simulink model "simple_high_fidelity_tilting_quadrotor_test"  (R2022b)
settings: Solver=ode4  StartTime=0.0  StopTime=10.0  FixedStep=T_s  RelTol=1e-3
undefined symbols (not defined in the file): alpha_0, N, w_bar_0
libraries: slpidlib x2, uavutilslib x1
settings Model: PauseTimes=0.2  Creator=pozzan  LastModifiedBy=pozzan

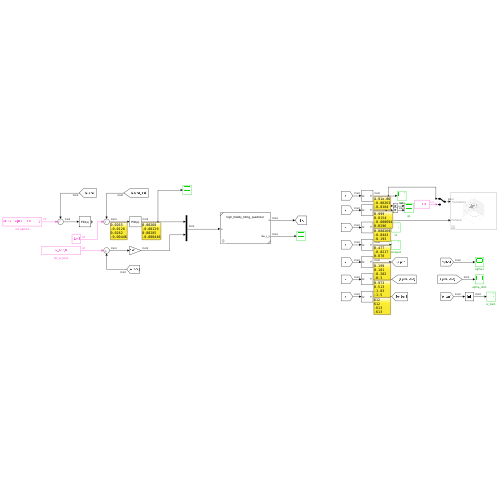
[thumbnail: Simulink's stored preview of the top-level diagram]
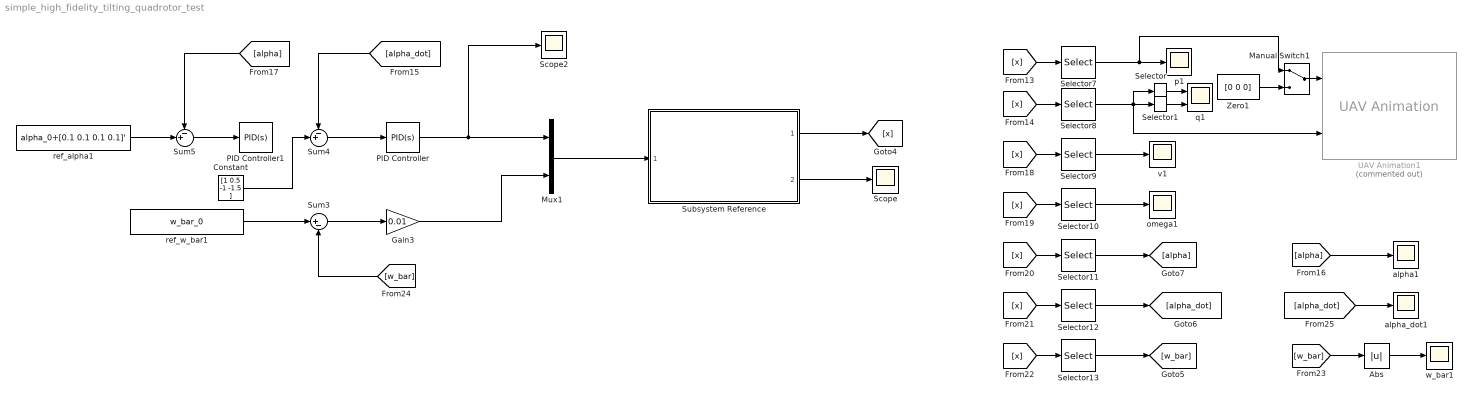
== system simple_high_fidelity_tilting_quadrotor_test ==
  Abs : Abs  SaturateOnIntegerOverflow=off
  Constant : Constant  Value=[1 0.5 -1 -1.5 ]
  Gain3 : Gain  Gain=0.01
  Manual Switch1 : ManualSwitch
  Mux1 : Mux  Inputs=2
  PID Controller : slpidlib/PID Controller  Controller=PID  Form=Parallel  TimeDomain=Continuous-time  UseExternalTs=off  SampleTime=-1  IntegratorMethod=Forward Euler  FilterMethod=Forward Euler  ControllerParametersSource=internal  P=0.1  I=0  UseKiTs=off  D=0.0001  N=100  UseFilter=on  TunerSelectOption=Transfer Function Based (PID Tuner App)  InitialConditionSource=internal  InitialConditionForIntegrator=0  InitialConditionForFilter=0  DifferentiatorICPrevScaledInput=0  ExternalReset=none  TrackingMode=off  Kt=1  LimitOutput=off  SatLimitsSource=internal  UpperSaturationLimit=inf  LowerSaturationLimit=-inf  LinearizeAsGain=on  AntiWindupMode=none  Kb=1  LimitIntegrator=off  UpperIntegratorSaturationLimit=inf  LowerIntegratorSaturationLimit=-inf  POutMin=[]  POutMax=[]  IOutMin=[]  IOutMax=[]  DOutMin=[]  DOutMax=[]  NOutMin=[]  NOutMax=[]  SumOutMin=[]  SumOutMax=[]  SaturationOutMin=[]  SaturationOutMax=[]  PParamMin=[]  PParamMax=[]  IParamMin=[]  IParamMax=[]  DParamMin=[]  DParamMax=[]  NParamMin=[]  NParamMax=[]  KbParamMin=[]  KbParamMax=[]  KtParamMin=[]  KtParamMax=[]  KbOutMin=[]  KbOutMax=[]  KtOutMin=[]  KtOutMax=[]  IntegratorOutMin=[]  IntegratorOutMax=[]  FilterOutMin=[]  FilterOutMax=[]  SumI1OutMin=[]  SumI1OutMax=[]  SumI2OutMin=[]  SumI2OutMax=[]  SumI3OutMin=[]  SumI3OutMax=[]  SumI4OutMin=[]  SumI4OutMax=[]  SumDOutMin=[]  SumDOutMax=[]  DifferentiatorOutMin=[]  DifferentiatorOutMax=[]  FilterDiffOutCoefMin=[]  FilterDiffOutCoefMax=[]  ReciprocalOutMin=[]  ReciprocalOutMax=[]  SumDenOutMin=[]  SumDenOutMax=[]  SumNumOutMin=[]  SumNumOutMax=[]  DivideOutMin=[]  DivideOutMax=[]  UdiffTsProdOutMin=[]  UdiffTsProdOutMax=[]  NTsProdOutMin=[]  NTsProdOutMax=[]  UintegralTsProdOutMin=[]  UintegralTsProdOutMax=[]  UngainTsProdOutMin=[]  UngainTsProdOutMax=[]  ClampingZeroOutDataTypeStr=Inherit: Inherit via back propagation  ClampingZeroOutMin=[]  ClampingZeroOutMax=[]  FilterDenConstantOutDataTypeStr=Inherit: Inherit via back propagation  FilterDenConstantOutMin=[]  FilterDenConstantOutMax=[]  PCopyOutDataTypeStr=Inherit: Inherit via back propagation  PCopyOutMin=[]  PCopyOutMax=[]  NCopyOutDataTypeStr=Inherit: Inherit via back propagation  NCopyOutMin=[]  NCopyOutMax=[]  IntegratorContinuousStateAttributes=''  IntegratorStateMustResolveToSignalObject=off  IntegratorRTWStateStorageClass=Auto  FilterContinuousStateAttributes=''  FilterStateMustResolveToSignalObject=off  FilterRTWStateStorageClass=Auto  ParallelPVariant=InternalParameters  IdealPVariant=Disabled  IVariant=InternalParameters  DVariant=InternalParameters  IntegratorVariant=Continuous  SatVariant=Disabled  AWVariant=Passthrough  PCopyVariant=Disabled  TRVariant=Disabled  FdbkBlocksVariant=Forward  IdealPFdbkVariant=Disabled  SatFdbkVariant=Disabled  DerivativeFilterVariant=ContFilter  NVariant=InternalParameters  NCopyVariant=Disabled  FilterICVariant=InternalICsFilter  IntegratorICVariant=InternalICs  ExternalResetVariant=Disabled  TRSumVariant=Passthrough  SumFdbkVariant=Disabled  SumVariant=Sum_PID  TsampFilterVariant=InternalTs  TsampNgainVariant=Passthrough  TsampIntegralVariant=Passthrough  ExternalSaturationOutDataTypeStr=Inherit: Same as second input
  PID Controller1 : slpidlib/PID Controller  Controller=PID  Form=Parallel  TimeDomain=Continuous-time  UseExternalTs=off  SampleTime=-1  IntegratorMethod=Forward Euler  FilterMethod=Forward Euler  ControllerParametersSource=internal  P=0.1  I=1  UseKiTs=off  D=0  N=100  UseFilter=on  TunerSelectOption=Transfer Function Based (PID Tuner App)  InitialConditionSource=internal  InitialConditionForIntegrator=0  InitialConditionForFilter=0  DifferentiatorICPrevScaledInput=0  ExternalReset=none  TrackingMode=off  Kt=1  LimitOutput=off  SatLimitsSource=internal  UpperSaturationLimit=inf  LowerSaturationLimit=-inf  LinearizeAsGain=on  AntiWindupMode=none  Kb=1  LimitIntegrator=off  UpperIntegratorSaturationLimit=inf  LowerIntegratorSaturationLimit=-inf  POutMin=[]  POutMax=[]  IOutMin=[]  IOutMax=[]  DOutMin=[]  DOutMax=[]  NOutMin=[]  NOutMax=[]  SumOutMin=[]  SumOutMax=[]  SaturationOutMin=[]  SaturationOutMax=[]  PParamMin=[]  PParamMax=[]  IParamMin=[]  IParamMax=[]  DParamMin=[]  DParamMax=[]  NParamMin=[]  NParamMax=[]  KbParamMin=[]  KbParamMax=[]  KtParamMin=[]  KtParamMax=[]  KbOutMin=[]  KbOutMax=[]  KtOutMin=[]  KtOutMax=[]  IntegratorOutMin=[]  IntegratorOutMax=[]  FilterOutMin=[]  FilterOutMax=[]  SumI1OutMin=[]  SumI1OutMax=[]  SumI2OutMin=[]  SumI2OutMax=[]  SumI3OutMin=[]  SumI3OutMax=[]  SumI4OutMin=[]  SumI4OutMax=[]  SumDOutMin=[]  SumDOutMax=[]  DifferentiatorOutMin=[]  DifferentiatorOutMax=[]  FilterDiffOutCoefMin=[]  FilterDiffOutCoefMax=[]  ReciprocalOutMin=[]  ReciprocalOutMax=[]  SumDenOutMin=[]  SumDenOutMax=[]  SumNumOutMin=[]  SumNumOutMax=[]  DivideOutMin=[]  DivideOutMax=[]  UdiffTsProdOutMin=[]  UdiffTsProdOutMax=[]  NTsProdOutMin=[]  NTsProdOutMax=[]  UintegralTsProdOutMin=[]  UintegralTsProdOutMax=[]  UngainTsProdOutMin=[]  UngainTsProdOutMax=[]  ClampingZeroOutDataTypeStr=Inherit: Inherit via back propagation  ClampingZeroOutMin=[]  ClampingZeroOutMax=[]  FilterDenConstantOutDataTypeStr=Inherit: Inherit via back propagation  FilterDenConstantOutMin=[]  FilterDenConstantOutMax=[]  PCopyOutDataTypeStr=Inherit: Inherit via back propagation  PCopyOutMin=[]  PCopyOutMax=[]  NCopyOutDataTypeStr=Inherit: Inherit via back propagation  NCopyOutMin=[]  NCopyOutMax=[]  IntegratorContinuousStateAttributes=''  IntegratorStateMustResolveToSignalObject=off  IntegratorRTWStateStorageClass=Auto  FilterContinuousStateAttributes=''  FilterStateMustResolveToSignalObject=off  FilterRTWStateStorageClass=Auto  ParallelPVariant=InternalParameters  IdealPVariant=Disabled  IVariant=InternalParameters  DVariant=InternalParameters  IntegratorVariant=Continuous  SatVariant=Disabled  AWVariant=Passthrough  PCopyVariant=Disabled  TRVariant=Disabled  FdbkBlocksVariant=Forward  IdealPFdbkVariant=Disabled  SatFdbkVariant=Disabled  DerivativeFilterVariant=ContFilter  NVariant=InternalParameters  NCopyVariant=Disabled  FilterICVariant=InternalICsFilter  IntegratorICVariant=InternalICs  ExternalResetVariant=Disabled  TRSumVariant=Passthrough  SumFdbkVariant=Disabled  SumVariant=Sum_PID  TsampFilterVariant=InternalTs  TsampNgainVariant=Passthrough  TsampIntegralVariant=Passthrough  ExternalSaturationOutDataTypeStr=Inherit: Same as second input
  Scope : Scope
  Scope2 : Scope
  Selector : Selector  InputPortWidth=4  IndexOptions=Index vector (dialog)  Indices=1  OutputSizes=1
  Selector1 : Selector  InputPortWidth=4  IndexOptions=Index vector (dialog)  Indices=2:4  OutputSizes=1
  Selector10 : Selector  InputPortWidth=13+3*N  IndexOptions=Index vector (dialog)  Indices=11:13  OutputSizes=1
  Selector11 : Selector  InputPortWidth=13+3*N  IndexOptions=Index vector (dialog)  Indices=14:14+N-1  OutputSizes=1
  Selector12 : Selector  InputPortWidth=13+3*N  IndexOptions=Index vector (dialog)  Indices=14+N:14+2*N-1  OutputSizes=1
  Selector13 : Selector  InputPortWidth=13+3*N  IndexOptions=Index vector (dialog)  Indices=14+2*N:14+3*N-1  OutputSizes=1
  Selector7 : Selector  InputPortWidth=13+3*N  IndexOptions=Index vector (dialog)  Indices=1:3  OutputSizes=1
  Selector8 : Selector  InputPortWidth=13+3*N  IndexOptions=Index vector (dialog)  Indices=4:7  OutputSizes=1
  Selector9 : Selector  InputPortWidth=13+3*N  IndexOptions=Index vector (dialog)  Indices=8:10  OutputSizes=1
  Subsystem Reference : Subsystem  ReferencedSubsystem=high_fidelity_tilting_quadrotor  p0=p_0  q0=q_0  v0=v_0  omega0=omega_0  alpha0=alpha_0  d_alpha_0=alpha_dot_0  bar_w0=w_bar_0  m_b=m_b  beta=beta  I_b=I_b  I_i=I_i  c_direction=c_direction  k_m=k_m  k_t=k_t  p_mot=p_mot
  Sum3 : Sum  Inputs=|+-
  Sum4 : Sum  Inputs=-+|
  Sum5 : Sum  Inputs=-+|
  UAV Animation1 : uavutilslib/UAV Animation  Commented=on  UAVType=Multirotor  UAVSize=1  InertialZDirection=Up  SampleTime=0.02
  Zero1 : Constant  Value=[0 0 0]  OutDataTypeStr=Inherit: Inherit via back propagation
  alpha1 : Scope
  alpha_dot1 : Scope
  omega1 : Scope
  p1 : Scope
  q1 : Scope  NumInputPorts=2
  ref_alpha1 : Constant  Value=alpha_0+[0.1 0.1 0.1 0.1]'  VectorParams1D=off
  ref_w_bar1 : Constant  Value=w_bar_0
  v1 : Scope
  w_bar1 : Scope
  wires:
  Selector10/1 -> omega1/1
  [w_bar] -> Abs/1
  Abs/1 -> w_bar1/1
  [x] -> Selector10/1
  [x] -> Selector11/1
  Zero1/1 -> Manual Switch1/2
  Selector13/1 -> [w_bar]
  [x] -> Selector7/1
  Selector12/1 -> [alpha_dot]
  Manual Switch1/1 -> UAV Animation1/1
  Selector9/1 -> v1/1
  [x] -> Selector8/1
  Selector11/1 -> [alpha]
  [alpha] -> alpha1/1
  Selector7/1 -> Manual Switch1/1, p1/1
  [alpha_dot] -> alpha_dot1/1
  Selector8/1 -> Selector1/1, Selector/1, UAV Animation1/2
  [x] -> Selector9/1
  [x] -> Selector12/1
  [x] -> Selector13/1
  Subsystem Reference/1 -> [x]
  Subsystem Reference/2 -> Scope/1
  PID Controller/1 -> Scope2/1, Mux1/1
  ref_w_bar1/1 -> Sum3/1
  [w_bar] -> Sum3/2
  Gain3/1 -> Mux1/2
  Mux1/1 -> Subsystem Reference/1
  Sum4/1 -> PID Controller/1
  Constant/1 -> Sum4/2
  Sum3/1 -> Gain3/1
  Sum5/1 -> PID Controller1/1
  [alpha_dot] -> Sum4/1
  [alpha] -> Sum5/1
  ref_alpha1/1 -> Sum5/2
  Selector/1 -> q1/1
  Selector1/1 -> q1/2
